simulink model "nomotoTransferFucntion"  (R2022b)
settings: Solver=VariableStepAuto  StartTime=0.0  StopTime=1900  RelTol=1e-3
undefined symbols (not defined in the file or in its folder): Iz, Kp, Kphi, Kr, Krrr, Kv, Kvrr, Kvvphi, Kvvr, Kvvv, lx, m, Np, Nphi, Nr, Nrrr, Nv, Nvrr, Nvvphi, Nvvr, Nvvv, Waypoints, Xphiphi, Xrr, Xrv, Xu, Xudot, Xuu, Xuuu, Xvv, Yp, Yphi, Yr, Yrrr, Yv, Yvrr, Yvvr, Yvvv
settings Model: Creator=ruben  LastModifiedBy=ruben
settings SolverCC: ZeroCrossAlgorithm=Adaptive
settings DebuggingCC: AlgebraicLoopMsg=none  UnderspecifiedInitializationDetection=Classic  IgnoredZcDiagnostic=none

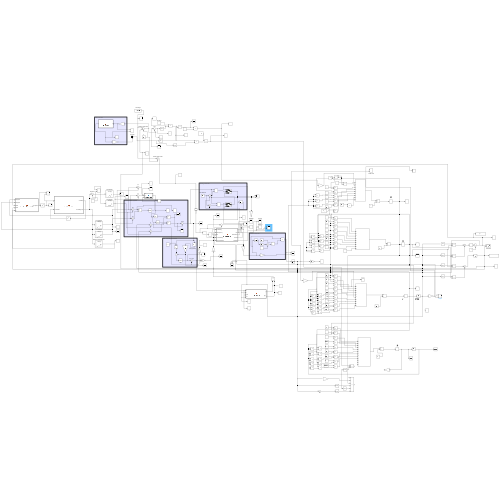
[thumbnail: Simulink's stored preview of the top-level diagram]
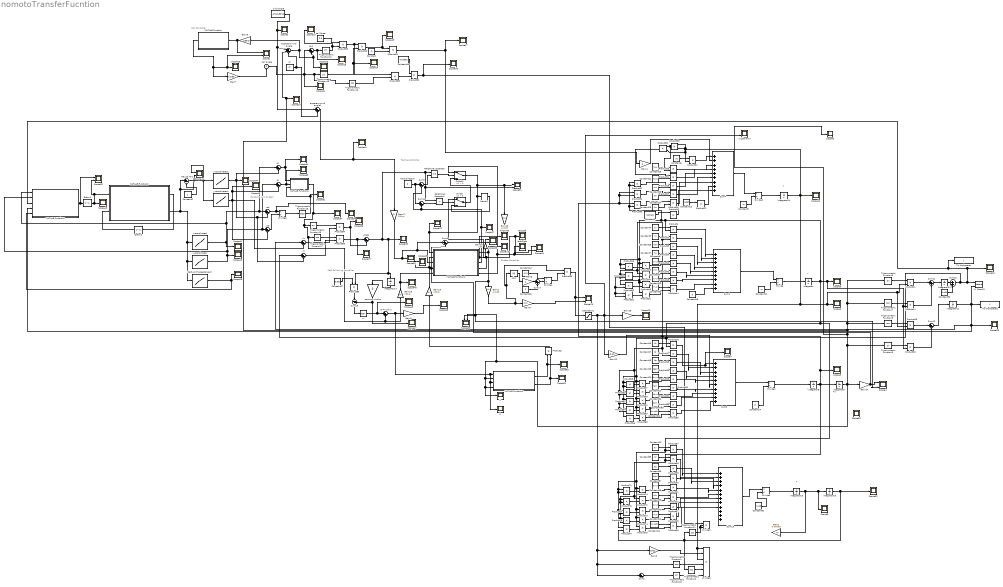
== system nomotoTransferFucntion ==
  note: Path Following Controller
  note: Guidance Axis System
  note: Sail Controller
  note: Tacking Controller
  note: Rudder Controller
  note: V
  note: r
  note: PSI
  note: U
  note: p
  Abs : Abs  SaturateOnIntegerOverflow=off
  AoA : Sum  Inputs=|++
  Constant : Constant  Value=-1
  Constant1 : Constant  Value=Xphiphi
  Constant10 : Constant  Value=Kv
  Constant11 : Constant  Value=m
  Constant12 : Constant  Value=-0.1
  Constant13 : Constant  Value=Xudot
  Constant14 : Constant  Value=Iz
  Constant15 : Constant  Value=Xuu
  Constant16 : Constant  Value=Nv
  Constant17 : Constant  Value=Nr
  Constant18 : Constant  Value=Np
  Constant19 : Constant  Value=Nphi
  Constant2 : Constant
  Constant20 : Constant  Value=Nvvv
  Constant21 : Constant  Value=Nrrr
  Constant22 : Constant  Value=Xuuu
  Constant23 : Constant  Value=Xvv
  Constant24 : Constant  Value=Xrr
  Constant25 : Constant  Value=Xrv
  Constant26 : Constant
  Constant27 : Constant  Value=0.001
  Constant28 : Constant  Value=Yphi
  Constant29 : Constant  Value=Yvvr
  Constant3 : Constant  Value=m
  Constant30 : Constant  Value=Yvrr
  Constant31 : Constant  Value=lx/10
  Constant32 : Constant  Value=Nvvr
  Constant33 : Constant  Value=Nvrr
  Constant34 : Constant  Value=Nvvphi
  Constant35 : Constant  Value=Kr
  Constant36 : Constant  Value=Kp
  Constant37 : Constant  Value=Kphi
  Constant38 : Constant  Value=Kvvv
  Constant39 : Constant  Value=Krrr
  Constant4 : Constant  Value=Yv
  Constant40 : Constant  Value=Kvvr
  Constant41 : Constant  Value=Kvrr
  Constant42 : Constant  Value=Kvvphi
  Constant43 : Constant  Value=-0.0001
  Constant45 : Constant  Value=0
  Constant5 : Constant  Value=Yr
  Constant50 : Constant  Value=-1401
  Constant6 : Constant  Value=Xu
  Constant7 : Constant  Value=Yp
  Constant8 : Constant  Value=Yvvv
  Constant9 : Constant  Value=Yrrr
  Delay1 : Delay  DelayLength=1  SampleTime=1
  Delay2 : Delay  DelayLength=1  SampleTime=1
  Divide{,1..4,6} (6 alike) : Product  Inputs=*/
  Divide5 : Product  Inputs=***
  Divide8 : Product  Inputs=******
  Gain1 : Gain  Gain=-0.00005
  Gain10 : Gain  Gain=100
  Gain{8..9,11,13..15,18} (7 alike) : Gain  Gain=180/pi
  Gain12 : Gain  Gain=-0.01
  Gain19 : Gain  Gain=pi/180
  Gain2 : Gain  Gain=pi/180
  Gain3 : Gain  Gain=0.001
  Gain4 : Gain
  Gain5 : Gain
  Gain6 : Gain  Gain=-0.1
  Gain7 : Gain  Gain=pi/180
  Integrator{,10..11,15} (4 alike) : Integrator
  Integrator14 : Integrator  InitialCondition=4  LowerSaturationLimit=0
  Integrator16 : Integrator  WrappedStateUpperValue=2*pi  WrappedStateLowerValue=0
  Integrator17 : Integrator  LimitOutput=on  UpperSaturationLimit=10  LowerSaturationLimit=-10
  Integrator8 : Integrator  UpperSaturationLimit=0.1  LowerSaturationLimit=-0.1
  Integrator9 : Integrator  WrappedStateUpperValue=2*pi  WrappedStateLowerValue=0
  MATLAB Function : MATLAB Function  TreatAsAtomicUnit=on
  MATLAB Function1 : MATLAB Function  TreatAsAtomicUnit=on
  MATLAB Function2 : MATLAB Function  TreatAsAtomicUnit=on
  MATLAB Function3 : MATLAB Function  TreatAsAtomicUnit=on
  MATLAB Function4 : MATLAB Function  TreatAsAtomicUnit=on
  MATLAB Function6 : MATLAB Function  TreatAsAtomicUnit=on
  Memory : Memory
  Product1 : Product  Inputs=3
  Product{2,6..81,84..85,88} (80 alike) : Product
  Radius of Acceptance R : Lookup_n-D  NumberOfTableDimensions=1  BreakpointsForDimension1=Waypoints.number  Table=Waypoints.R  InterpMethod=Cubic spline  ExtrapMethod=Cubic spline  InternalRulePriority=Speed  RndMeth=Simplest
  Relational Operator : RelationalOperator  Operator=<=  OutDataTypeStr=boolean  RndMeth=Simplest  InputSameDT=off
  Relational Operator1 : RelationalOperator  Operator=>  OutDataTypeStr=boolean  RndMeth=Simplest  InputSameDT=off
  Saturation1 : Saturate  UpperLimit=0.3  LowerLimit=-0.3
  Scope{1,4,13,19,31,46,50,52..54} (10 alike) : Scope  NumInputPorts=2
  Scope{2..3,5..7,9..12,14..18,20..30,32..45,47..49,51,58,63..65} (47 alike) : Scope
  Scope8 : Scope  NumInputPorts=3
  Sum1 : Sum  Inputs=|+++++++++
  Sum{11,14..15,17} (4 alike) : Sum  Inputs=|++
  Sum{2..3,5,12} (4 alike) : Sum  Inputs=|+-
  Sum13 : Sum  Inputs=|++++++++++++
  Sum16 : Sum  Inputs=|--
  Sum4 : Sum  Inputs=|+++++++++
  Sum9 : Sum  Inputs=|++++++++++
  Switch : Switch  Criteria=u2 > Threshold  SaturateOnIntegerOverflow=off  InputSameDT=off
  Switch1 : Switch  Criteria=u2 > Threshold  SaturateOnIntegerOverflow=off  InputSameDT=off
  TACKING : Scope
  Tack Direction : Constant  Value=0
  To Workspace : ToWorkspace  VariableName=x  SaveFormat=Timeseries  SampleTime=-1
  To Workspace1 : ToWorkspace  VariableName=y  SaveFormat=Timeseries  SampleTime=-1
  Trigonometric Function{1..2,7..8,10..11,17} (7 alike) : Trigonometry  Operator=cos
  Trigonometric Function{3,6,9,12..13,16} (6 alike) : Trigonometry
  Trigonometric Function15 : Trigonometry  Operator=atan
  U : Scope
  V : Scope
  Waypoint-1 : Sum  Inputs=|+-
  XY Graph3 : Record  FileSettingsInternal="{\"entries\":[{\"content\":{\"excelSettings\":{\"content\":{},\"type\":\"Streamout.ExcelSettings\"}},\"type\":\"Streamout.FileSettingStorage\",\"uuid\":\"938be52b-556f-40b6-b0e9-ec3a9bb5bd26\"}],\"packageUris\":[\"http://schema.mathworks.com/mf0/streamout_blocks/R2020a\"],\"version\":\"1.0\"}"  Layout=[1 1]  SignalsInternal="{\"entries\":[{\"content\":{\"signals\":[{\"content\":{\"blockPath\":[\"nomotoTransferFucntion/XY Graph3\"],\"channel\":[],\"dimensions\":[1],\"domain\":\"nomotoTransferFucntion/XY Graph3\",\"lineColor\":\"#0072bd\",\"plots\":[],\"port\":1,\"sid\":[\"\"],\"signalID\":526,\"signalName\":\"Sum15\"},\"type\":\"RecordBlkView.Signal\",\"uuid\":\"83430481-853c-4a7d-a58a-5169d3bdf0e8\"},{\"content\":{\"blockPath\":[\"nomotoTransferFucntion/XY Graph3\"],\"channel\":[],\"dimensions\":[1],\"domain\":\"nomotoTransferFucntion/XY Graph3\",\"lineColor\":\"#d95319\",\"plots\":[],\"port\":2,\"sid\":[\"\"],\"signalID\":530,\"signalName\":\"Integrator11\"},\"type\":\"RecordBlkView.Signal\",\"uuid\":\"35e64786-a76e-4cf0-98cb-e07aee4450e2\"}]},\"type\":\"RecordBlkView.InputSignals\",\"uuid\":\"8067bf04-9257-4b02-945f-13205029dc6c\"}],\"packageUris\":[\"http://schema.mathworks.com/mf0/streamout_blocks/R2020a\"],\"version\":\"1.0\"}"  VisualizationBindings="{\"xyplotplugin\":{\"info\":[{\"series\":[],\"subplotID\":1}]}}"  CompatibilityTag=XY
  apparent wind angle : Sum  Inputs=|-+-
  apparent wind angle1 : Sum  Inputs=|++
  causing windup : Gain  Gain=0
  pi : Constant  Value=pi
  qx : Sum  Inputs=|+-
  qy : Sum  Inputs=|+-
  rudder anhl : Scope  NumInputPorts=2
  sail angle : Sum  Inputs=|+
  sail force : Constant  Value=2.5
  tackLeft : Scope
  tackRight : Scope
  wind angle : Constant  Value=-170/180*pi  VectorParams1D=off
  x-coordinates : Lookup_n-D  NumberOfTableDimensions=1  BreakpointsForDimension1=Waypoints.number  Table=Waypoints.x  InterpMethod=Cubic spline  ExtrapMethod=Cubic spline  InternalRulePriority=Speed  RndMeth=Simplest
  x-coordinates1 : Lookup_n-D  NumberOfTableDimensions=1  BreakpointsForDimension1=Waypoints.number  Table=Waypoints.x  InterpMethod=Cubic spline  ExtrapMethod=Cubic spline  InternalRulePriority=Speed  RndMeth=Simplest
  xd = xp+xr : Sum  Inputs=|++
  xh : Sum  Inputs=|+-
  xr : Trigonometry  Operator=atan
  xsd : Sum  Inputs=|+-
  y-coordinates : Lookup_n-D  NumberOfTableDimensions=1  BreakpointsForDimension1=Waypoints.number  Table=Waypoints.y  InterpMethod=Cubic spline  ExtrapMethod=Cubic spline  InternalRulePriority=Speed  RndMeth=Simplest
  y-coordinates1 : Lookup_n-D  NumberOfTableDimensions=1  BreakpointsForDimension1=Waypoints.number  Table=Waypoints.y  InterpMethod=Cubic spline  ExtrapMethod=Cubic spline  InternalRulePriority=Speed  RndMeth=Simplest
  yh : Sum  Inputs=|+-
  ysd : Sum  Inputs=|+-
  ytrack : Sum  Inputs=|+-
  wires:
  Constant4/1 -> Product6/1
  Constant5/1 -> Product7/1
  Constant7/1 -> Product9/1
  Constant8/1 -> Product10/1
  Constant9/1 -> Product42/1
  Product6/1 -> Sum1/1
  Product7/1 -> Sum1/2
  Product8/1 -> Sum1/3
  Product9/1 -> Sum1/4
  Product10/1 -> Sum1/5
  Product42/1 -> Sum1/6
  Sum1/1 -> Divide/1
  Divide/1 -> Integrator/1
  Constant11/1 -> Divide/2
  Product16/1 -> Scope7/1, Sum9/1
  Constant18/1 -> Product18/1
  Product18/1 -> Sum9/3
  Product19/1 -> Sum9/4
  Constant16/1 -> Product16/1
  Product13/1 -> Sum9/5
  Constant14/1 -> Divide1/2
  Product17/1 -> Sum9/2
  Sum9/1 -> Divide1/1
  Constant17/1 -> Product17/1
  Trigonometric Function6/1 -> Product11/1
  Trigonometric Function7/1 -> Product14/1
  Product11/1 -> Sum11/1
  Product14/1 -> Sum11/2
  Sum11/1 -> Integrator10/1
  Product15/1 -> Sum12/1
  Sum12/1 -> Integrator11/1
  Trigonometric Function8/1 -> Product15/1
  Trigonometric Function9/1 -> Product20/1
  Product20/1 -> Sum12/2
  Constant20/1 -> Product13/1
  Sum4/1 -> Divide2/1
  Constant3/1 -> Divide2/2
  Divide2/1 -> Integrator14/1
  Product21/1 -> Sum4/1
  Constant6/1 -> Product21/1
  Constant13/1 -> Product22/1
  Constant19/1 -> Product19/1
  Gain4/1 -> Sum4/2
  Product25/1 -> Sum4/3
  Product24/1 -> Sum4/4
  Product26/1 -> Sum4/5
  Constant22/1 -> Product24/2
  Constant15/1 -> Product25/1
  Constant23/1 -> Product26/2
  Product22/1 -> Sum4/8
  Product27/1 -> Sum4/6
  Product28/1 -> Sum4/7
  Constant24/1 -> Product27/2
  Constant25/1 -> Product28/2
  Product29/1 -> Product25/2, Product30/1
  Product30/1 -> Product24/1
  Product31/1 -> Product26/1
  Product32/1 -> Product27/1
  Product33/1 -> Product28/1
  sail force/1 -> Product35/1
  Trigonometric Function13/1 -> Product23/2, Scope14/1
  Trigonometric Function12/1 -> Scope12/1, Product35/2
  AoA/1 -> Scope15/1, Trigonometric Function12/1
  Product35/1 -> Product80/1, Product23/1
  Product23/1 -> Scope18/1, Product34/1
  Constant/1 -> Product34/2
  Integrator14/1 -> Product29/2, Product29/1, Product30/2, Product21/2, Scope11/1, Divide8/3, Divide8/1, Product15/2, Product11/2, Scope6/1
  sail angle/1 -> Scope24/1, AoA/1, Trigonometric Function10/1, Trigonometric Function13/1
  Sum17/1 -> Divide4/2
  Constant12/1 -> Divide4/1
  Divide4/1 -> Product36/2
  Gain5/1 -> Sum17/1
  Constant26/1 -> Sum17/2
  Abs/1 -> Gain5/1
  Gain7/1 -> sail angle/1
  Gain8/1 -> Scope1/1, MATLAB Function/1(u)
  Gain2/1 -> Gain6/1, Product36/1, Abs/1
  Product37/1 -> Sum13/1
  Product38/1 -> Sum13/2
  Product39/1 -> Sum13/3
  Product41/1 -> Sum13/5
  Constant28/1 -> Product8/1
  Constant29/1 -> Product43/1
  Product43/1 -> Sum1/7
  Product44/1 -> Sum1/8
  Sum13/1 -> Divide3/1
  Divide3/1 -> Integrator15/1
  Integrator15/1 -> Gain1/1, Scope9/1, Integrator16/1
  Product45/1 -> Product10/2
  Product46/1 -> Product45/2
  Product47/1 -> Product42/2
  Product48/1 -> Product47/2
  Product50/1 -> Product49/2
  Product49/1 -> Product43/2
  Constant30/1 -> Product44/1
  Product52/1 -> Product51/2
  Product51/1 -> Product44/2
  Constant31/1 -> Divide3/2
  Product53/1 -> Sum9/7
  Product54/1 -> Sum9/8
  Product55/1 -> Sum9/9
  Product56/1 -> Sum9/10
  Constant34/1 -> Product56/1
  Constant33/1 -> Product55/1
  Constant32/1 -> Product54/1
  Constant21/1 -> Product53/1
  Product57/1 -> Product13/2
  Product58/1 -> Product57/2
  Product59/1 -> Product53/2
  Product60/1 -> Product59/2
  Product62/1 -> Product61/2
  Product61/1 -> Product54/2
  Product64/1 -> Product63/2
  Product63/1 -> Product55/2
  Product66/1 -> Product65/2
  Product65/1 -> Product56/2
  Gain12/1 -> Sum9/6
  Product40/1 -> Sum13/4
  Product12/1 -> Sum13/6
  Product67/1 -> Sum13/7
  Product68/1 -> Sum13/8
  Product69/1 -> Sum13/9
  Constant10/1 -> Product37/1
  Constant35/1 -> Product38/1
  Constant36/1 -> Product39/1
  Constant37/1 -> Product40/1
  Constant38/1 -> Product41/1
  Constant39/1 -> Product12/1
  Constant40/1 -> Product67/1
  Constant41/1 -> Product68/1
  Constant42/1 -> Product69/1
  Product71/1 -> Product70/2
  Product76/1 -> Product72/2
  Product77/1 -> Product73/2
  Product78/1 -> Product74/2
  Product79/1 -> Product75/2
  Integrator8/1 -> Product78/2, Product78/1, Product77/2, Product76/2, Product76/1, Product72/1, Product38/2, Integrator9/1, Product64/1, Product64/2, Product62/2, Product60/2, Product60/1, Product59/1, Product17/2, Product33/1, Product32/2, Product32/1, Product52/2, Product52/1, Product50/2, Product48/2, Product48/1, Product47/1, Product7/2, Scope3/1
  Integrator/1 -> Product65/1, Product63/1, Product61/1, Product57/1, Product58/2, Product66/1, Product62/1, Product58/1, Product16/2, Product79/1, Product77/1, Product71/2, Product71/1, Product75/1, Product74/1, Product73/1, Product70/1, Product37/2, Product20/2, Product14/2, Scope5/1, Product33/2, Product31/2, Product31/1, Product50/1, Product51/1, Product49/1, Product45/1, Product46/2, Product46/1, Product6/2
  Trigonometric Function10/1 -> Product80/2
  Product80/1 -> Product81/2
  Constant43/1 -> Product81/1
  Product81/1 -> Scope33/1, Divide5/1
  Trigonometric Function11/1 -> Divide5/3, Divide5/2
  Product34/1 -> Scope17/1, Gain4/1
  Integrator16/1 -> Trigonometric Function2/1, Trigonometric Function11/1, Product79/2, Scope32/1
  xsd/1 -> Scope39/1, Divide6/1
  Product85/1 -> Scope37/1, ytrack/1
  ysd/1 -> Divide6/2
  Trigonometric Function17/1 -> Product85/1
  Product84/1 -> Scope36/1, ytrack/2
  Relational Operator1/1 -> Switch/2
  Relational Operator/1 -> Switch1/2
  Switch/1 -> Switch1/3
  Sum3/1 -> Relational Operator/2
  Sum14/1 -> Relational Operator1/2
  Tack Direction/1 -> Sum14/1, Sum3/1
  Integrator10/1 -> Sum15/1
  Constant50/1 -> Sum15/2
  Trigonometric Function15/1 -> Scope51/1, MATLAB Function6/3(u)
  Radius of Acceptance R/1 -> Scope28/1, MATLAB Function3/5(R)
  xr/1 -> Scope49/1, xd = xp+xr/1
  Trigonometric Function16/1 -> Product84/1
  Integrator11/1 -> MATLAB Function3/4(yBoat), Scope38/1, yh/1, To Workspace1/1, XY Graph3/2
  yh/1 -> Product84/2
  xh/1 -> Product85/2
  Integrator17/1 -> causing windup/1
  Sum16/1 -> xr/1
  Constant45/1 -> Sum1/9
  Divide1/1 -> Integrator8/1
  MATLAB Function/1(y) -> Gain7/1, Scope1/2, Scope26/1
  wind angle/1 -> Scope2/1, apparent wind angle1/1, apparent wind angle/1
  apparent wind angle/1 -> AoA/2, Scope23/1, Gain8/1
  Saturation1/1 -> Sum2/1, Trigonometric Function1/1, Gain3/1, Gain12/1, Gain18/1, rudder anhl/2
  Gain3/1 -> Divide8/2
  Trigonometric Function1/1 -> Divide8/4
  Trigonometric Function2/1 -> Divide8/5
  Trigonometric Function3/1 -> Divide8/6
  Sum2/1 -> Trigonometric Function3/1
  Product1/1 -> Sum4/9
  Constant1/1 -> Product1/1
  Product70/1 -> Product41/2
  Product72/1 -> Product12/2
  Product73/1 -> Product67/2
  Product74/1 -> Product68/2
  Product75/1 -> Product69/2
  Switch1/1 -> MATLAB Function1/1(tackHeading), Scope22/1, Memory/1, Gain19/1, Scope31/1
  apparent wind angle1/1 -> Scope40/1, Gain11/1
  pi/1 -> apparent wind angle/3, apparent wind angle1/2
  MATLAB Function2/2(currentWaypoint) -> Scope46/2, Waypoint-1/1, Radius of Acceptance R/1, y-coordinates/1, x-coordinates/1
  MATLAB Function2/1(nextState) -> Delay2/1
  Delay2/1 -> MATLAB Function2/2(currentState)
  x-coordinates/1 -> MATLAB Function3/1(xWaypoint), qx/1, xsd/1, Scope41/1
  y-coordinates/1 -> qy/1, ysd/1, MATLAB Function3/2(yWaypoint), Scope42/1
  Constant2/1 -> Waypoint-1/2
  MATLAB Function3/1(acceptance) -> Scope52/1, Delay1/1
  Gain9/1 -> Scope25/1
  Waypoint-1/1 -> y-coordinates1/1, Scope46/1, x-coordinates1/1
  y-coordinates1/1 -> qy/2, Scope45/1, yh/2, ysd/2
  ytrack/1 -> Product88/2, Integrator17/1, Scope35/1, Relational Operator1/1, Scope31/2, Relational Operator/1
  Divide6/1 -> Trigonometric Function15/1
  Product36/1 -> Saturation1/1, Scope19/1
  Delay1/1 -> Scope43/1, Scope52/2, MATLAB Function2/1(R)
  causing windup/1 -> Scope47/1, Sum16/2
  qy/1 -> Scope65/1, MATLAB Function6/2(y1)
  qx/1 -> MATLAB Function6/1(x1), Scope64/1
  MATLAB Function6/1(y) -> xd = xp+xr/2, Gain15/1, Trigonometric Function17/1, Trigonometric Function16/1, Scope34/1
  x-coordinates1/1 -> qx/2, Scope44/1, xsd/2, xh/2
  MATLAB Function1/1(y) -> Scope4/2, Scope50/1, Gain2/1, Scope10/1
  Gain18/1 -> Scope20/1
  Memory/1 -> Switch/3
  Gain6/1 -> Scope19/2
  Constant27/1 -> Product88/1
  Integrator9/1 -> Trigonometric Function6/1, Trigonometric Function7/1, Trigonometric Function8/1, apparent wind angle/2, Scope13/1, Scope8/2, Trigonometric Function9/1, Scope50/2, MATLAB Function4/2(v), V/1, MATLAB Function4/4(psi), Gain14/1
  MATLAB Function1/3(tackDistance) -> Scope27/1, Sum3/2, Sum14/2
  MATLAB Function4/1(y) -> Scope63/1, Product2/1
  Sum15/1 -> Scope16/1, To Workspace/1, MATLAB Function3/3(xBoat), XY Graph3/1, xh/1
  MATLAB Function1/2(tack) -> Gain10/1, TACKING/1
  MATLAB Function1/4(tackLeft) -> Switch/1, Scope54/1, tackLeft/1
  MATLAB Function1/5(tackRight) -> Scope54/2, tackRight/1, Switch1/1
  Gain13/1 -> MATLAB Function1/2(pathTrajectory), Scope29/1
  Gain15/1 -> MATLAB Function1/5(wayPointHeading), Scope48/1
  xd = xp+xr/1 -> Gain9/1, MATLAB Function4/1(u), U/1, MATLAB Function4/3(psid)
  MATLAB Function4/2(sign) -> Scope21/1, Product2/2
  Product2/1 -> Gain13/1
  Product88/1 -> Sum16/1
  Sum5/1 -> Scope53/2
  Gain11/1 -> Scope30/1, Sum5/1, MATLAB Function1/3(WA)
  Gain14/1 -> Sum5/2, MATLAB Function1/4(currentHeading), Scope4/1
  Gain10/1 -> Scope53/1

== matlab function nomotoTransferFucntion/MATLAB Function1 ==
  data: tackHeading input; pathTrajectory input; y output; WA input; tack output; currentHeading input; tackDistance output; tackLeft output; tackRight output; wayPointHeading input
function [y,tack,tackDistance,tackLeft,tackRight]  = headingController(tackHeading,pathTrajectory,WA,currentHeading,wayPointHeading)
% Change wind angle to follow same convection as waypoint heading, ranges
% from -180 -> 180
if WA<-180
    WA = WA + 360;
end
if WA>180
    WA = WA - 360;
end

% Determine the state of sailboat
if      abs(wayPointHeading-WA)<45
    % State 1: Tacking   
           % Initialize tacking right
           if(abs(tackHeading)<15)
                % Set tack angle to the right
                y=WA+45;
                % State value
                tack=0.5;
                % Tack Distance D
                tackDistance=100;
                % Tack Right Angle
                tackRight=WA+45;
                % Tack LEft Angle
                tackLeft=WA-45;
           else
               % Reference heading
               y=tackHeading-currentHeading;
               % State value
               tack=1;
               % Tack Right Angle
               tackRight=WA+45;
               % Tack LEft Angle
               tackLeft=WA-45;
               % Tack Distance D
               tackDistance=100;
           end
% State 0: Normal Sail 
else 
        % State Value
        tack=0;
        % Reference Heading
        y=pathTrajectory;
        % Reset tacking distance
        tackDistance=100;
        % Reset Right tack angle
        tackRight=45;
        % Reset Left tack angle
        tackLeft=-45;
end

== matlab function nomotoTransferFucntion/MATLAB Function ==
  data: u input; y output
function y = sailController(u)
% Convert apparent wind angle to the range 0 -> 360
if(u<360)
    % Sail control equation implementation
    if(u<180)
    y = -0.5*u;
    else
    y=-0.5*u+180;
    end
else
    % Sail control equation implementation
    u=u-360;
    if(u<180)
    y = -0.5*u;
    else
    y=-0.5*u+180;
    end
end
end

== matlab function nomotoTransferFucntion/MATLAB Function2 ==
  data: R input; nextState output; currentWaypoint output; currentState input
function [nextState,currentWaypoint]  = wayPointController(R,currentState)
% Waypoint switching
% With each added waypoint another case should be added
switch currentState
    % First waypoint
    case 0
        % Check if waypoint lies within radius of acceptance
        if(R==1)
            % Switch current Waypoint to next waypoint
            nextState=1;
            currentWaypoint=1;
        % Waypoint not reached
        else
            nextState=0;
            currentWaypoint=0;
        end
    case 1
        % Check if waypoint lies within radius of acceptance
        if(R==1)
            % Switch current Waypoint to next waypoint
            nextState=2;
            currentWaypoint=2;
       % Waypoint not reached
       else
            nextState=currentState;
            currentWaypoint=1;
       end
    case 2
       % Check if waypoint lies within radius of acceptance
       if(R==1)
            % Switch current Waypoint to next waypoint
            nextState=3;
            currentWaypoint=3;
       % Waypoint not reached
       else
            nextState=currentState;
            currentWaypoint=2;
       end
     case 3
       % Check if waypoint lies within radius of acceptance
       if(R==1)
            % Switch current Waypoint to next waypoint
            nextState=4;
            currentWaypoint=4;
       % Waypoint not reached 
       else
            nextState=currentState;
            currentWaypoint=3;
       end
     case 4
       % Check if waypoint lies within radius of acceptance
       if(R==1)
            % Switch current Waypoint to next waypoint
            nextState=0;
            currentWaypoint=0;
       % Waypoint not reached
       else
            nextState=currentState;
            currentWaypoint=4;
       end
    otherwise
        nextState=0;
        currentWaypoint=0;
end

== matlab function nomotoTransferFucntion/MATLAB Function3 ==
  data: xWaypoint input; yWaypoint input; xBoat input; yBoat input; R input; acceptance output
function acceptance   = circleOfAcceptanceController(xWaypoint,yWaypoint,xBoat,yBoat,R)
    if (sqrt((abs(xWaypoint-xBoat))^2+(abs(yWaypoint-yBoat))^2)<R)
        acceptance=1;
    else
        acceptance=0;
    end
end

== matlab function nomotoTransferFucntion/MATLAB Function4 ==
  data: u input; y output; v input; psid input; psi input; sign output
function [y,sign] = referenceAngle(u,v,psid,psi)
% Calculate vector components of desired heading
u1= sin(u);
u2 = cos(u);

% Calculate vetor components of actual heading
v1= sin(v);
v2 = cos(v);


if (psid<0)
    psid = psid +2*pi;
end
if psi< 0
 psi=psi+2*pi;
end 

if(psi-psid)>0
    sign=-1;
else 
    sign=1;
end
dotProduct = u1*v1 + u2*v2;
theta = acos(dotProduct);

y = theta;

== matlab function nomotoTransferFucntion/MATLAB Function6 ==
  data: x1 input; y1 input; u input; y output
function y = controlAngle(x1,y1,u)
if x1>=0 && y1>=0
    y=u;
elseif x1==0 && y1>0
        y=0;
elseif x1==0 && y1<0
        y=-pi;
elseif y1==0 && x1>0
        y=pi/2;
elseif y1==0 && x1<0
        y=pi/2;
elseif x1<0 && y1>0
    y=u;
elseif x1<0 && y1<0
    y=-pi+u;
else
    y=-pi+u;
end
